simulink model "sldemo_tc"  (R2024a)
settings: Solver=ode3  StartTime=0.0  StopTime=10.0  FixedStep=0.005  RelTol=1e-3
StartFcn:
  | set_param('sldemo_tc/Scope','Open','on')
undefined symbols (not defined in the file or in its folder): TypeS_bits_bp, TypeS_tdegc_interp, TypeS_tdegc_vs_bits
libraries: simulink_extras x1
Description:
  | Thermocouple Modeling and Signal Conversion
  | 
  | The thermocouple is one of the popular analog transducers today, along
  | with other devices such as position sensors, strain gages, pressure
  | transducers, and resistance temperature devices (RTDs). Operating under
  | the principle of the Seebeck (or thermoelectric) effect, thermocouples
  | have an empirically determined nonlinear behavior that is well known over
  | each junction type's useful operating range. If you run the model, you
  | will be able to see the cumulative effect of each component on dynamic
  | measurement accuracy. This demonstration will focus on models for each of
  | these components in a dynamic temperature measurement system for a Type S
  | (Platinum-10% Rhodium(+) versus Platinum(-) ) : a thermocouple device and
  | probe assembly, a signal conditioning method, an analog to digital
  | converter (ADC), and a software specification for converting the ADC
  | output back into a temperature value. An additional section shows how to
  | obtain and use standard NIST ITS-90 thermocouple data with Simulink
  | models. Look-up tables and a polynomial block are used in this design to
  | capture the nonlinear behavior of the thermocouple. Note that the
  | polynomial block is a viable alternative to look-up tables for some
  | applications, minimizing ROM usage at the cost of some additional
  | computation for the full polynomial representation.
settings Model: Creator=The MathWorks, Inc.  LastModifiedBy=neham
settings SolverCC: AlgebraicLoopSolver=TrustRegion
settings DataIOCC: LimitDataPoints=on  SaveFormat=Array  SaveOutput=off  SaveTime=off
settings OptimizationCC: DefaultParameterBehavior=Inlined  InlineInvariantSignals=on  ExpressionDepthLimit=2147483647  InitFltsAndDblsToZero=on  LifeSpan=inf  BufferReusableBoundary=off
settings DebuggingCC: SaveWithParameterizedLinksMsg=none  UnderspecifiedInitializationDetection=Classic  MergeDetectMultiDrivingBlocksExec=none  CheckExecutionContextPreStartOutputMsg=on  SignalResolutionControl=TryResolveAllWithWarning  SolverPrmCheckMsg=warning  MultiTaskDSMMsg=warning  MultiTaskCondExecSysMsg=none  FcnCallInpInsideContextMsg=warning  UnconnectedInputMsg=warning  UnconnectedOutputMsg=warning  UnconnectedLineMsg=warning  BusObjectLabelMismatch=none  StateNameClashWarn=warning  SFUnexpectedBacktrackingDiag=warning  SFNoUnconditionalDefaultTransitionDiag=warning  SFExecutionAtInitializationDiag=none  ArithmeticOperatorsInVariantConditions=warning
settings HardwareCC: ProdBitPerPointer=32  ProdBitPerSizeT=32  ProdBitPerPtrDiffT=32  ProdLargestAtomicFloat=None  ProdIntDivRoundTo=Floor  ProdWordSize=32  ProdHWDeviceType=32-bit xPC Target (AMD Athlon)
settings ModelReferenceCC: EnableRefExpFcnMdlSchedulingChecks=on  PropagateSignalLabelsOutOfModel=off
settings SFSimCC: SimUseLocalCustomCode=off  CustomCodeUndefinedFunction=UseInterfaceOnly
settings RTWCC: GenCodeOnly=on  RTWUseLocalCustomCode=off  GPUComputeCapability=3.5
settings CodeAppCC: StateflowObjectComments=on
settings GRTTargetCC: TargetFcnLib=iso_tfl_tmw.mat  CombineOutputUpdateFcns=off  GRTInterface=on
settings ConfigComp: CovMetricSettings=dw  CovSaveCumulativeToWorkspaceVar=on  CovSaveSingleToWorkspaceVar=on  CovExternalEMLEnable=off

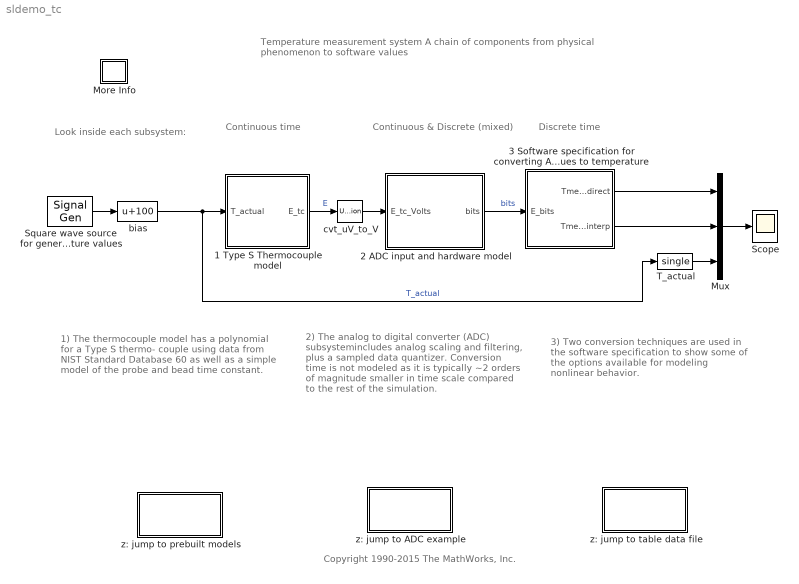
== system sldemo_tc ==
  note: Temperature measurement system
      | A chain of components from
      | physical phenomenon to software values
  note: 1) The thermocouple model has
      | a polynomial for a Type S thermo-
      | couple using data from NIST
      | Standard Database 60 as well
      | as a simple model of the probe
      | and bead time constant.
  note: 2) The analog to digital converter
      | (ADC) subsystemincludes analog
      | scaling and filtering, plus a
      | sampled data quantizer.
      | Conversion time is not modeled
      | as it is typically ~2 orders of
      | magnitude smaller in time scale
      | compared to the rest of the
      | simulation.
  note: 3) Two conversion techniques
      | are used  in the software
      | specification to show some
      | of the options available for
      | modeling nonlinear behavior.
  note: Continuous
      | time
  note: Discrete
      | time
  note: Continuous &
      | Discrete (mixed)
  note: Look inside
      | each subsystem:
  note: Copyright 1990-2015 The MathWorks, Inc.
  1 Type S Thermocouple model : Subsystem
  2 ADC input and hardware model : Subsystem
  3 Software specification for converting ADC values to temperature : Subsystem
  More Info : Subsystem
      settings: OpenFcn=showExample('simulink_general/sldemo_tc_scriptExample')
      mask Display: disp('?')
  Mux : Mux  Inputs=3
  Scope : Scope
  Square wave source for generating temperature values : SignalGenerator  WaveForm=square  Amplitude=100
  T_actual : DataTypeConversion  OutDataTypeStr=single  SaturateOnIntegerOverflow=off  RndMeth=Floor
  bias : Bias  Bias=100  SaturateOnIntegerOverflow=off
  cvt_uV_to_V : UnitConversion
  z: jump to ADC example : Subsystem  mask(ADC quantizer details){}
      mask help: Jump to a model that exercises more details of the behavior of the Idealized ADC quantizer block that is part of the hardware model.
      settings: OpenFcn=open_system('sldemo_adc_quantize','force')
      mask Display: disp('ADC Quantizer\nDetails')
  z: jump to prebuilt models : Subsystem  mask(ADC quantizer details){}
      mask help: Jump to a model that exercises more details of the behavior of the Idealized ADC quantizer block that is part of the hardware model.
      settings: OpenFcn=open_system('sldemo_tc_blocks','force')
      mask Display: disp('Additional\nThermocouple\nModels')
  z: jump to table data file : Subsystem  mask(ADC quantizer details){}
      mask help: Jump to a model that exercises more details of the behavior of the Idealized ADC quantizer block that is part of the hardware model.
      settings: OpenFcn=edit sldemo_create_tc_tabledata.m
      mask Display: disp('Table Design\nDetails')
  wires:
  3 Software specification for converting ADC values to temperature/1(Tmeas_direct) -> Mux/1
  1 Type S Thermocouple model/1(E_tc) -> cvt_uV_to_V/1  "E"
  2 ADC input and hardware model/1(bits) -> 3 Software specification for converting ADC values to temperature/1(E_bits)  "bits"
  3 Software specification for converting ADC values to temperature/2(Tmeas_interp) -> Mux/2
  Mux/1 -> Scope/1
  bias/1 -> 1 Type S Thermocouple model/1(T_actual), T_actual/1  "T_actual"
  Square wave source for generating temperature values/1 -> bias/1
  T_actual/1 -> Mux/3
  cvt_uV_to_V/1 -> 2 ADC input and hardware model/1(E_tc_Volts)

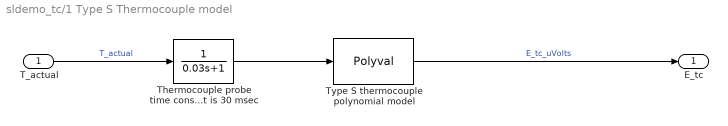
== system sldemo_tc/1 Type S Thermocouple model ==
  T_actual : Inport  Unit=degC
  Thermocouple probe time constant is 30 msec : TransferFcn  Denominator=[0.03 1]
  Type S thermocouple polynomial model : Polyval  Description=|  Coefs=[ +2.71443176145e-021, -1.25068871393e-017, +2.55744251786e-014, -3.31465196389e-011, +3.22028823036e-008, -2.32477968689e-005, +1.25934289740e-002, +5.40313308631e+000, +0.00000000000e+000 ]
      | 0 deg C ice reference         
      |       microVolts = f(Temperature degC)   
      | (Segment 1) input range: -50 to 1063 degC
      settings: AttributesFormatString=%<Description>
  E_tc : Outport  Unit=uV  VectorParamsAs1DForOutWhenUnconnected=off
  wires:
  Thermocouple probe time constant is 30 msec/1 -> Type S thermocouple polynomial model/1
  T_actual/1 -> Thermocouple probe time constant is 30 msec/1  "T_actual"
  Type S thermocouple polynomial model/1 -> E_tc/1  "E_tc_uVolts"

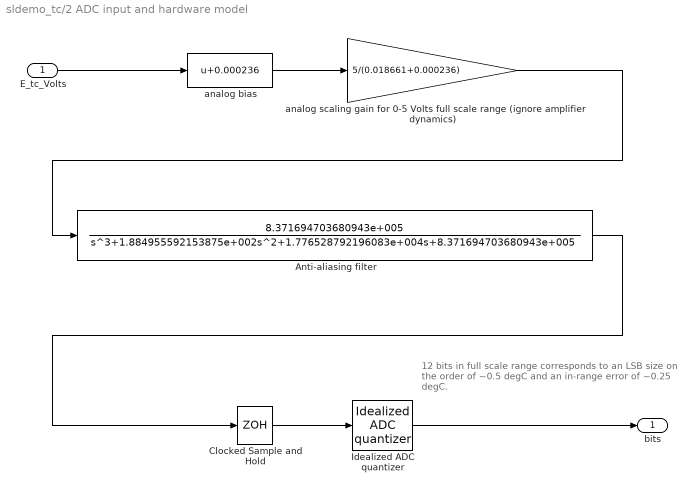
== system sldemo_tc/2 ADC input and hardware model ==
  note: 12 bits in full scale range corresponds to
      | an LSB size on the order of ~0.5 degC and
      | an in-range error of ~0.25 degC.
  E_tc_Volts : Inport  Unit=V
  Anti-aliasing filter : TransferFcn  Description=|  Numerator=8.371694703680943e+005  Denominator=[ 1, 1.884955592153875e+002, 1.776528792196083e+004, 8.371694703680943e+005 ]
      | Designed using Signal Processing Toolbox command:
      | >> [num,den] = butter(3,15*2*pi,'low','s')
      settings: AttributesFormatString=%<Description>
  Clocked Sample and Hold : ZeroOrderHold  SampleTime=0.020
      settings: AttributesFormatString=(%<SampleTime> sec)
  Idealized ADC quantizer : simulink_extras/Additional Discrete/Idealized ADC quantizer  NumberOfConverterBits=12  Vmin=0  Vmax=5  OutputDataType=uint16  OutputNegativeValues=off
      settings: SourceProductName=Simulink
  analog bias : Bias  Bias=0.000236  SaturateOnIntegerOverflow=off
  analog scaling gain for 0-5 Volts full scale range (ignore amplifier dynamics) : Gain  Gain=5/(0.018661+0.000236)
  bits : Outport  Unit=count  VectorParamsAs1DForOutWhenUnconnected=off
  wires:
  analog scaling gain for 0-5 Volts full scale range (ignore amplifier dynamics)/1 -> Anti-aliasing filter/1
  E_tc_Volts/1 -> analog bias/1
  Clocked Sample and Hold/1 -> Idealized ADC quantizer/1
  Idealized ADC quantizer/1 -> bits/1
  analog bias/1 -> analog scaling gain for 0-5 Volts full scale range (ignore amplifier dynamics)/1
  Anti-aliasing filter/1 -> Clocked Sample and Hold/1

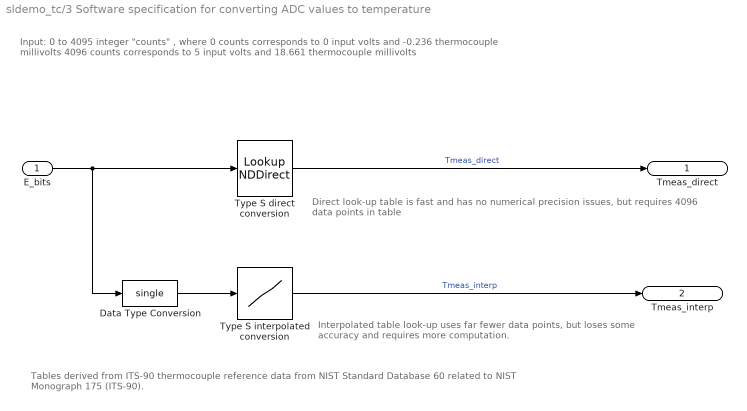
== system sldemo_tc/3 Software specification for converting ADC values to temperature ==
  note: Input: 0 to 4095 integer "counts" , where
      |             0        counts corresponds to 0 input volts and -0.236 thermocouple millivolts
      |             4096 counts corresponds to 5 input volts and 18.661 thermocouple millivolts
  note: Tables derived from ITS-90 thermocouple reference data
      | from NIST Standard Database 60 related to NIST Monograph 175 (ITS-90).
  note: Direct look-up table is fast and has no numerical precision issues,
      | but requires 4096 data points in table
  note: Interpolated table look-up uses far fewer data points,
      | but loses some accuracy and requires more computation.
  E_bits : Inport  OutDataTypeStr=uint16  Unit=count
  Data Type Conversion : DataTypeConversion  OutDataTypeStr=single  SaturateOnIntegerOverflow=off  RndMeth=Floor
  Type S direct conversion : LookupNDDirect  NumberOfTableDimensions=1  Table=TypeS_tdegc_vs_bits
      settings: AttributesFormatString=(%<mxTable>)
  Type S interpolated conversion : Lookup_n-D  NumberOfTableDimensions=1  BreakpointsForDimension1=TypeS_bits_bp  IndexSearchMethod=Linear search  BeginIndexSearchUsingPreviousIndexResult=on  Table=TypeS_tdegc_interp  ExtrapMethod=Clip  DiagnosticForOutOfRangeInput=Warning  InternalRulePriority=Speed  RndMeth=Simplest
      settings: AttributesFormatString=(%<tableData>)
  Tmeas_direct : Outport  Unit=degC  VectorParamsAs1DForOutWhenUnconnected=off
  Tmeas_interp : Outport  Port=2  Unit=degC  VectorParamsAs1DForOutWhenUnconnected=off
  wires:
  E_bits/1 -> Type S direct conversion/1, Data Type Conversion/1
  Type S direct conversion/1 -> Tmeas_direct/1  "Tmeas_direct"
  Data Type Conversion/1 -> Type S interpolated conversion/1
  Type S interpolated conversion/1 -> Tmeas_interp/1  "Tmeas_interp"

== system sldemo_tc/More Info ==

== system sldemo_tc/z: jump to ADC example ==
  note: This block intentionally has no contents.

== system sldemo_tc/z: jump to prebuilt models ==
  note: This block intentionally has no contents.

== system sldemo_tc/z: jump to table data file ==
  note: This block intentionally has no contents.
